simulink model "dds_cwg"  (R2016b)
(part 10 of 67)

      mask prompts: io_names "Names [msb...lsb]"; io_widths "Bitwidths [msb...lsb]"; io_bps "Binary pts [msb...lsb]"; io_types "Data types [msb...lsb], ufix=0, fix=1, bool=2"; show_format "Print format string?"; snap_storage "Storage medium"; snap_dram_dimm "DRAM dimm"; snap_dram_clock "DRAM clock rate"; snap_nsamples "Number of Samples (2^?)"; snap_data_width "Data width"; snap_offset "Start delay support"; snap_circap "Circular capture support"; snap_value "Extra value capture support"; snap_ext_arm "External arm support"; snap_ext_circ "External circular capture support"; snap_provide_outputs "Provide outputs"; snap_use_dsp48 "Use DSP48s to implement counters"; snap_delay "Pre-snapshot delay"; extra_names "Names [msb...lsb]"; extra_widths "Widths [msb...lsb]"; extra_bps "Binary pts [msb...lsb]"; extra_types "Data types [msb...lsb], ufix=0, fix=1, bool=2"
      mask help:
      | A wrapped snapshot block. Allows specification of inputs to a snapblock word so the toolflow can automatically set up the scope.
      | See documentation for snapshot for explanation of parameters.
      mask init:
      | bitsnap_init(gcb);
      settings: AttributesFormatString=|
      | snap(3):f10.9,b,b = 12 bits\n16 wide, 8192 deep
      | debugID: 72770927
      mask TypeOptions snap_storage: bram | dram
      mask Callback snap_storage: bitsnap_callback();
      mask TypeOptions snap_dram_dimm: 1 | 2 | 3 | 4
      mask TypeOptions snap_dram_clock: 200 | 250 | 266 | 300 | 333
      mask TypeOptions snap_data_width: 8 | 16 | 32 | 64 | 128
      mask Callback snap_value: bitsnap_callback();
      mask Callback snap_ext_arm: bitsnap_callback();
      mask Callback snap_ext_circ: bitsnap_callback();
      mask Callback snap_provide_outputs: bitsnap_callback();
  ss_fir_out : Subsystem  Tag=casper:bitsnap  Commented=on  AncestorBlock=casper_library_scopes/bitfield_snapshot  mask(bitsnap){io_names=[fir sync dv], io_widths=[18 1 1], io_bps=[17 0 0], io_types=[1 2 2], show_format=on, snap_storage=bram, snap_dram_dimm=2, snap_dram_clock=250, snap_nsamples=13, snap_data_width=32, snap_offset=off, snap_circap=off, snap_value=off, snap_ext_arm=off, snap_ext_circ=off, snap_provide_outputs=on, snap_use_dsp48=on, snap_delay=2, extra_names=timestamp, extra_widths=32, extra_bps=0, extra_types=0}
      mask prompts: io_names "Names [msb...lsb]"; io_widths "Bitwidths [msb...lsb]"; io_bps "Binary pts [msb...lsb]"; io_types "Data types [msb...lsb], ufix=0, fix=1, bool=2"; show_format "Print format string?"; snap_storage "Storage medium"; snap_dram_dimm "DRAM dimm"; snap_dram_clock "DRAM clock rate"; snap_nsamples "Number of Samples (2^?)"; snap_data_width "Data width"; snap_offset "Start delay support"; snap_circap "Circular capture support"; snap_value "Extra value capture support"; snap_ext_arm "External arm support"; snap_ext_circ "External circular capture support"; snap_provide_outputs "Provide outputs"; snap_use_dsp48 "Use DSP48s to implement counters"; snap_delay "Pre-snapshot delay"; extra_names "Names [msb...lsb]"; extra_widths "Widths [msb...lsb]"; extra_bps "Binary pts [msb...lsb]"; extra_types "Data types [msb...lsb], ufix=0, fix=1, bool=2"
      mask help:
      | A wrapped snapshot block. Allows specification of inputs to a snapblock word so the toolflow can automatically set up the scope.
      | See documentation for snapshot for explanation of parameters.
      mask init:
      | bitsnap_init(gcb);
      settings: AttributesFormatString=|
      | snap(3):f18.17,b,b = 20 bits\n32 wide, 8192 deep
      | debugID: 20209532
      mask TypeOptions snap_storage: bram | dram
      mask Callback snap_storage: bitsnap_callback();
      mask TypeOptions snap_dram_dimm: 1 | 2 | 3 | 4
      mask TypeOptions snap_dram_clock: 200 | 250 | 266 | 300 | 333
      mask TypeOptions snap_data_width: 8 | 16 | 32 | 64 | 128
      mask Callback snap_value: bitsnap_callback();
      mask Callback snap_ext_arm: bitsnap_callback();
      mask Callback snap_ext_circ: bitsnap_callback();
      mask Callback snap_provide_outputs: bitsnap_callback();
  ss_fir_out1 : Subsystem  Tag=casper:bitsnap  AncestorBlock=casper_library_scopes/bitfield_snapshot  mask(bitsnap){io_names=[fir sync dv], io_widths=[18 1 1], io_bps=[17 0 0], io_types=[1 2 2], show_format=on, snap_storage=bram, snap_dram_dimm=2, snap_dram_clock=250, snap_nsamples=13, snap_data_width=32, snap_offset=off, snap_circap=off, snap_value=off, snap_ext_arm=off, snap_ext_circ=off, snap_provide_outputs=on, snap_use_dsp48=on, snap_delay=2, extra_names=timestamp, extra_widths=32, extra_bps=0, extra_types=0}
      mask prompts: io_names "Names [msb...lsb]"; io_widths "Bitwidths [msb...lsb]"; io_bps "Binary pts [msb...lsb]"; io_types "Data types [msb...lsb], ufix=0, fix=1, bool=2"; show_format "Print format string?"; snap_storage "Storage medium"; snap_dram_dimm "DRAM dimm"; snap_dram_clock "DRAM clock rate"; snap_nsamples "Number of Samples (2^?)"; snap_data_width "Data width"; snap_offset "Start delay support"; snap_circap "Circular capture support"; snap_value "Extra value capture support"; snap_ext_arm "External arm support"; snap_ext_circ "External circular capture support"; snap_provide_outputs "Provide outputs"; snap_use_dsp48 "Use DSP48s to implement counters"; snap_delay "Pre-snapshot delay"; extra_names "Names [msb...lsb]"; extra_widths "Widths [msb...lsb]"; extra_bps "Binary pts [msb...lsb]"; extra_types "Data types [msb...lsb], ufix=0, fix=1, bool=2"
      mask help:
      | A wrapped snapshot block. Allows specification of inputs to a snapblock word so the toolflow can automatically set up the scope.
      | See documentation for snapshot for explanation of parameters.
      mask init:
      | bitsnap_init(gcb);
      settings: AttributesFormatString=|
      | snap(3):f18.17,b,b = 20 bits\n32 wide, 8192 deep
      | debugID: 89618929
      mask TypeOptions snap_storage: bram | dram
      mask Callback snap_storage: bitsnap_callback();
      mask TypeOptions snap_dram_dimm: 1 | 2 | 3 | 4
      mask TypeOptions snap_dram_clock: 200 | 250 | 266 | 300 | 333
      mask TypeOptions snap_data_width: 8 | 16 | 32 | 64 | 128
      mask Callback snap_value: bitsnap_callback();
      mask Callback snap_ext_arm: bitsnap_callback();
      mask Callback snap_ext_circ: bitsnap_callback();
      mask Callback snap_provide_outputs: bitsnap_callback();
  ss_nb : Subsystem  Tag=casper:bitsnap  AncestorBlock=casper_library_scopes/bitfield_snapshot  mask(bitsnap){io_names=[r0 i0 r1 i1 sync dv sync_cnt], io_widths=[18 18 18 18 1 1 11], io_bps=[17 17 17 17 0 0 0], io_types=[1 1 1 1 2 2 0], show_format=on, snap_storage=bram, snap_dram_dimm=2, snap_dram_clock=250, snap_nsamples=9, snap_data_width=128, snap_offset=off, snap_circap=off, snap_value=off, snap_ext_arm=off, snap_ext_circ=off, snap_provide_outputs=on, snap_use_dsp48=on, snap_delay=2, extra_names=timestamp, extra_widths=32, extra_bps=0, extra_types=0}
      mask prompts: io_names "Names [msb...lsb]"; io_widths "Bitwidths [msb...lsb]"; io_bps "Binary pts [msb...lsb]"; io_types "Data types [msb...lsb], ufix=0, fix=1, bool=2"; show_format "Print format string?"; snap_storage "Storage medium"; snap_dram_dimm "DRAM dimm"; snap_dram_clock "DRAM clock rate"; snap_nsamples "Number of Samples (2^?)"; snap_data_width "Data width"; snap_offset "Start delay support"; snap_circap "Circular capture support"; snap_value "Extra value capture support"; snap_ext_arm "External arm support"; snap_ext_circ "External circular capture support"; snap_provide_outputs "Provide outputs"; snap_use_dsp48 "Use DSP48s to implement counters"; snap_delay "Pre-snapshot delay"; extra_names "Names [msb...lsb]"; extra_widths "Widths [msb...lsb]"; extra_bps "Binary pts [msb...lsb]"; extra_types "Data types [msb...lsb], ufix=0, fix=1, bool=2"
      mask help:
      | A wrapped snapshot block. Allows specification of inputs to a snapblock word so the toolflow can automatically set up the scope.
      | See documentation for snapshot for explanation of parameters.
      mask init:
      | bitsnap_init(gcb);
      settings: AttributesFormatString=|
      | snap(7):f18.17,f18.17,f18.17,f18.17,b,b,uf11.0 = 85 bits\n128 wide, 512 deep
      | debugID: 83317040
      mask TypeOptions snap_storage: bram | dram
      mask Callback snap_storage: bitsnap_callback();
      mask TypeOptions snap_dram_dimm: 1 | 2 | 3 | 4
      mask TypeOptions snap_dram_clock: 200 | 250 | 266 | 300 | 333
      mask TypeOptions snap_data_width: 8 | 16 | 32 | 64 | 128
      mask Callback snap_value: bitsnap_callback();
      mask Callback snap_ext_arm: bitsnap_callback();
      mask Callback snap_ext_circ: bitsnap_callback();
      mask Callback snap_provide_outputs: bitsnap_callback();
  ss_nb1 : Subsystem  Tag=casper:bitsnap  AncestorBlock=casper_library_scopes/bitfield_snapshot  mask(bitsnap){io_names=[r2 i2 r3 i3 sync dv sync_cnt], io_widths=[18 18 18 18 1 1 11], io_bps=[17 17 17 17 0 0 0], io_types=[1 1 1 1 2 2 0], show_format=on, snap_storage=bram, snap_dram_dimm=2, snap_dram_clock=250, snap_nsamples=9, snap_data_width=128, snap_offset=off, snap_circap=off, snap_value=off, snap_ext_arm=off, snap_ext_circ=off, snap_provide_outputs=on, snap_use_dsp48=on, snap_delay=2, extra_names=timestamp, extra_widths=32, extra_bps=0, extra_types=0}
      mask prompts: io_names "Names [msb...lsb]"; io_widths "Bitwidths [msb...lsb]"; io_bps "Binary pts [msb...lsb]"; io_types "Data types [msb...lsb], ufix=0, fix=1, bool=2"; show_format "Print format string?"; snap_storage "Storage medium"; snap_dram_dimm "DRAM dimm"; snap_dram_clock "DRAM clock rate"; snap_nsamples "Number of Samples (2^?)"; snap_data_width "Data width"; snap_offset "Start delay support"; snap_circap "Circular capture support"; snap_value "Extra value capture support"; snap_ext_arm "External arm support"; snap_ext_circ "External circular capture support"; snap_provide_outputs "Provide outputs"; snap_use_dsp48 "Use DSP48s to implement counters"; snap_delay "Pre-snapshot delay"; extra_names "Names [msb...lsb]"; extra_widths "Widths [msb...lsb]"; extra_bps "Binary pts [msb...lsb]"; extra_types "Data types [msb...lsb], ufix=0, fix=1, bool=2"
      mask help:
      | A wrapped snapshot block. Allows specification of inputs to a snapblock word so the toolflow can automatically set up the scope.
      | See documentation for snapshot for explanation of parameters.
      mask init:
      | bitsnap_init(gcb);
      settings: AttributesFormatString=|
      | snap(7):f18.17,f18.17,f18.17,f18.17,b,b,uf11.0 = 85 bits\n128 wide, 512 deep
      | debugID: 32685757
      mask TypeOptions snap_storage: bram | dram
      mask Callback snap_storage: bitsnap_callback();
      mask TypeOptions snap_dram_dimm: 1 | 2 | 3 | 4
      mask TypeOptions snap_dram_clock: 200 | 250 | 266 | 300 | 333
      mask TypeOptions snap_data_width: 8 | 16 | 32 | 64 | 128
      mask Callback snap_value: bitsnap_callback();
      mask Callback snap_ext_arm: bitsnap_callback();
      mask Callback snap_ext_circ: bitsnap_callback();
      mask Callback snap_provide_outputs: bitsnap_callback();
  tlast_sel : Subsystem  Tag=xps:sw_reg  AncestorBlock=xps_library/Memory/software_register  mask(swreg){io_dir=From Processor, io_delay=0, init_val=0, sample_period=1, names=[sel], bitwidths=[1], bin_pts=0, arith_types=2, sim_port=on, show_format=on}
      mask prompts: io_dir "I/O direction"; io_delay "I/O delay"; init_val "Initial Value"; sample_period "Sample period"; names "Bitfield names [msb...lsb]"; bitwidths "Bitfield widths"; bin_pts "Bitfield binary pts"; arith_types "Bitfield types, ufix=0, fix=1, bool=2"; sim_port "Provide sim input/output?"; show_format "Print format string?"
      mask help: A 32-bit software-accessible register. Can be divided into bitfields of varying widths and types using the fields in the block mask.
      mask init:
      | swreg_init(gcb)
      settings: AttributesFormatString=1input:b = 1 bits
      mask TypeOptions io_dir: To Processor | From Processor
      mask Callback io_dir:
      | mask_enables = get_param(gcb, 'MaskEnables');
      | mask_names = get_param(gcb, 'MaskNames');
      | if strcmp(get_param(gcb, 'io_dir'), 'To Processor'),
      |     mask_enables{ismember(mask_names, 'sample_period')} = 'off';
      | else
      |     mask_enables{ismember(mask_names, 'sample_period')} = 'on';
      | end
      | set_param(gcb, 'MaskEnables', mask_enables);
      mask DialogControl ParameterTabVar0 Prompt: Setup
  tready_sel : Subsystem  Tag=xps:sw_reg  AncestorBlock=xps_library/Memory/software_register  mask(swreg){io_dir=From Processor, io_delay=0, init_val=0, sample_period=1, names=[sel], bitwidths=[1], bin_pts=0, arith_types=2, sim_port=on, show_format=on}
      mask prompts: io_dir "I/O direction"; io_delay "I/O delay"; init_val "Initial Value"; sample_period "Sample period"; names "Bitfield names [msb...lsb]"; bitwidths "Bitfield widths"; bin_pts "Bitfield binary pts"; arith_types "Bitfield types, ufix=0, fix=1, bool=2"; sim_port "Provide sim input/output?"; show_format "Print format string?"
      mask help: A 32-bit software-accessible register. Can be divided into bitfields of varying widths and types using the fields in the block mask.
      mask init:
      | swreg_init(gcb)
      settings: AttributesFormatString=1input:b = 1 bits
      mask TypeOptions io_dir: To Processor | From Processor
      mask Callback io_dir:
      | mask_enables = get_param(gcb, 'MaskEnables');
      | mask_names = get_param(gcb, 'MaskNames');
      | if strcmp(get_param(gcb, 'io_dir'), 'To Processor'),
      |     mask_enables{ismember(mask_names, 'sample_period')} = 'off';
      | else
      |     mask_enables{ismember(mask_names, 'sample_period')} = 'on';
      | end
      | set_param(gcb, 'MaskEnables', mask_enables);
      mask DialogControl ParameterTabVar0 Prompt: Setup
  tvalid_sel : Subsystem  Tag=xps:sw_reg  AncestorBlock=xps_library/Memory/software_register  mask(swreg){io_dir=From Processor, io_delay=0, init_val=0, sample_period=1, names=[sel], bitwidths=[1], bin_pts=0, arith_types=2, sim_port=on, show_format=on}
      mask prompts: io_dir "I/O direction"; io_delay "I/O delay"; init_val "Initial Value"; sample_period "Sample period"; names "Bitfield names [msb...lsb]"; bitwidths "Bitfield widths"; bin_pts "Bitfield binary pts"; arith_types "Bitfield types, ufix=0, fix=1, bool=2"; sim_port "Provide sim input/output?"; show_format "Print format string?"
      mask help: A 32-bit software-accessible register. Can be divided into bitfields of varying widths and types using the fields in the block mask.
      mask init:
      | swreg_init(gcb)
      settings: AttributesFormatString=1input:b = 1 bits
      mask TypeOptions io_dir: To Processor | From Processor
      mask Callback io_dir:
      | mask_enables = get_param(gcb, 'MaskEnables');
      | mask_names = get_param(gcb, 'MaskNames');
      | if strcmp(get_param(gcb, 'io_dir'), 'To Processor'),
      |     mask_enables{ismember(mask_names, 'sample_period')} = 'off';
      | else
      |     mask_enables{ismember(mask_names, 'sample_period')} = 'on';
      | end
      | set_param(gcb, 'MaskEnables', mask_enables);
      mask DialogControl ParameterTabVar0 Prompt: Setup
  sync_out : Outport
  pol0_out : Outport  Port=2
  pol1_out : Outport  Port=3
  dv_out : Outport  Port=4
  tag scope: capture_now=global, conf_tvalid=global, current_channel=global, data_pol0=global, data_tlast=global, data_trdy=global, fft_ch0=global, fft_ch1=global, fft_ch2=global, fft_dv0=global, fft_dv1=global, fft_dv2=global, fft_dvalid=global, fft_sync=global, fft_sync_count=global, fft_tl0=global, fft_tl1=global, fft_tl2=global, fft_tready_p0=global, fft_tready_p1=global, fft_tready_p2=global, fir_data_tlast=global, fir_dvalid_pol0=global, fir_pol0=global, fir_sync=global
  wires:
  From51/1 -> Delay13/1
  From49/1 -> Delay11/1
  Fast Fourier Transform 9.0 1/1 -> Terminator19/1
  Reinterpret1/1 -> Concat/2
  [fft_re_pol0] -> Gateway Out26/1
  Gateway Out54/1 -> To Workspace54/1
  From27/1 -> Gateway Out55/1
  Gateway Out52/1 -> To Workspace51/1
  From28/1 -> Gateway Out56/1
  pfb_fir_generic/2(pol0_out0) -> pipeline18/1(d)
  pfb_fir_generic/3(dvalid) -> pipeline19/1(d)
  pfb_fir_generic1/2(pol0_out0) -> pipeline20/1(d)
  pfb_fir_generic/1(sync_out) -> pipeline17/1(d)
  pfb_fir_generic1/1(sync_out) -> Terminator5/1
  Gateway Out56/1 -> To Workspace57/1
  Gateway Out55/1 -> To Workspace56/1
  Gateway Out26/1 -> To Workspace34/1
  Gateway Out37/1 -> To Workspace37/1
  Gateway Out38/1 -> To Workspace38/1
  pfb_fir_generic1/3(dvalid) -> pipeline21/1(d)
  [fft_fs0] -> Gateway Out54/1
  [fft_im_pol0] -> Gateway Out37/1
  Reinterpret/1 -> Concat/1
  [fft_tl0] -> Gateway Out38/1
  Reinterpret2/1 -> Concat3/1
  Reinterpret3/1 -> Concat3/2
  Concat3/1 -> Goto4/1
  Gateway Out18/1 -> To Workspace19/1
  Register11/1 -> bus_expand7/1(bus_in), Delay26/1
  Register10/1 -> Delay25/1
  Register9/1 -> Delay23/1
  Register1/1 -> bus_expand6/1(bus_in), Delay22/1
  Concat/1 -> [data_pol0]
  [capture_now] -> Register1/3
  [capture_now] -> Register9/3
  [capture_now] -> Register10/3
  [capture_now] -> Register11/3
  pipeline9/1(q) -> [fft_tl0]
  pol1/1 -> pfb_fir_generic1/2(pol0_in0)
  pipeline18/1(q) -> [fir_pol0], Gateway Out4/1
  pipeline20/1(q) -> [fir_pol1]
  Gateway Out3/1 -> To Workspace3/1
  pipeline17/1(q) -> [fir_sync], Gateway Out6/1
  Gateway Out7/1 -> To Workspace7/1
  Gateway Out16/1 -> To Workspace16/1
  [fft_sync] -> Gateway Out16/1
  pipeline8/1(q) -> [fft_dv0]
  [fft_dvalid] -> Gateway Out3/1
  [fft_tready_p0] -> Gateway Out52/1
  Gateway Out21/1 -> To Workspace21/1
  bus_expand1/1(msb_out8) -> Gateway Out21/1
  Gateway Out23/1 -> To Workspace23/1
  bus_expand1/2(out7) -> Gateway Out23/1
  Gateway Out24/1 -> To Workspace24/1
  bus_expand1/3(out6) -> Gateway Out24/1
  Gateway Out25/1 -> To Workspace27/1
  bus_expand1/4(out5) -> Gateway Out25/1
  Gateway Out28/1 -> To Workspace25/1
  bus_expand1/5(out4) -> Gateway Out28/1
  Gateway Out29/1 -> To Workspace28/1
  bus_expand1/6(out3) -> Gateway Out29/1
  Gateway Out30/1 -> To Workspace26/1
  bus_expand1/7(out2) -> Gateway Out30/1
  Gateway Out31/1 -> To Workspace29/1
  bus_expand1/8(lsb_out1) -> Gateway Out31/1
  Delay19/1 -> Register9/1
  Delay20/1 -> Register10/1
  Gateway Out6/1 -> To Workspace6/1
  Gateway Out1/1 -> To Workspace1/1
  Gateway Out4/1 -> To Workspace4/1
  Gateway Out15/1 -> To Workspace15/1
  Gateway Out33/1 -> To Workspace31/1
  Gateway Out34/1 -> To Workspace32/1
  pipeline28/1(q) -> [fft0_data_in_ch_halt]
  pipeline27/1(q) -> [fft0_event_tlast_miss]
  pipeline25/1(q) -> [fft0_event_tlast_unexp]
  [fft0_event_tlast_miss] -> Gateway Out15/1
  [fft0_event_tlast_unexp] -> Gateway Out33/1
  Gateway Out9/1 -> To Workspace9/1
  Gateway Out36/1 -> To Workspace36/1
  Gateway Out39/1 -> To Workspace39/1
  Delay3/1 -> Delay9/1
  Delay4/1 -> Delay8/1
  Gateway Out40/1 -> To Workspace40/1
  edge_detect3/1(out) -> [fft_sync]
  pipeline10/1(q) -> [fft_ch0]
  Concat5/1 -> pipeline45/1(d)
  [fft_ch] -> Gateway Out78/1, Delay12/1, Relational1/1, Delay18/1, Relational2/1
  [current_channel] -> Gateway Out34/1
  [current_channel] -> Relational/1, Delay5/1
  lsb_1/1 -> Logical6/2, Logical4/2
  lsb_0/1 -> Logical6/1, Logical4/1
  Logical4/1 -> edge_detect2/1
  [fft_dvalid] -> Delay1/1
  edge_detect2/1 -> Gateway Out40/1, [capture_now]
  [capture_now] -> Delay10/1
  Delay10/1 -> Gateway Out61/1, Delay32/1
  Register4/1 -> Concat1/4
  Register3/1 -> Concat1/3
  Register5/1 -> Concat1/2
  Register2/1 -> Concat1/1
  From1/1 -> Register2/3
  From33/1 -> Register5/3
  From34/1 -> Register3/3
  From36/1 -> Register4/3
  pipeline3/1(q) -> Register5/1
  pipeline4/1(q) -> Register3/1
  From14/1 -> Register2/2, Register5/2, Register3/2, Register4/2
  Delay13/1 -> Reinterpret3/1
  Delay11/1 -> Reinterpret2/1
  Register6/1 -> Delay16/1, Delay19/1, Delay20/1, bus_expand4/1(bus_in), Register11/1
  Delay1/1 -> Gateway Out76/1, Logical4/3
  pipeline2/1(q) -> Register2/1
  Constant/1 -> Relational/2
  Relational/1 -> Gateway Out41/1, Logical4/4
  Gateway Out41/1 -> To Workspace41/1
  pipeline44/1(q) -> [fft_fs0]
  Register12/1 -> Register4/1, pipeline4/1(d), pipeline3/1(d), pipeline2/1(d)
  From43/1 -> Register12/1
  From15/1 -> Delay7/1
  Delay7/1 -> Register12/2
  Concat1/1 -> pipeline47/1(d)
  pipeline45/1(q) -> bus_expand1/1(bus_in), pol1_out/1, bus_expand2/1(bus_in), pol0_out/1
  pipeline46/1(q) -> dv_out/1, Gateway Out18/1, pipeline80/1(d), pipeline68/1(d), pipeline82/1(d), pipeline70/1(d), Counter1/2
  pipeline19/1(q) -> Gateway Out1/1, [fir_dvalid_pol0]
  pipeline21/1(q) -> [fir_dvalid_pol1]
  pipeline26/1(q) -> [fft_tready_p0]
  pipeline13/1(q) -> [fft0_status_ch_halt]
  pipeline14/1(q) -> [fft0_data_out_ch_halt]
  Gateway Out10/1 -> To Workspace10/1
  [fft0_data_in_ch_halt] -> Gateway Out10/1
  Gateway Out11/1 -> To Workspace11/1
  [fft0_status_ch_halt] -> Gateway Out11/1
  Gateway Out42/1 -> To Workspace42/1
  [fft0_data_out_ch_halt] -> Gateway Out42/1
  Fast Fourier Transform 9.0 2/1 -> Terminator1/1
  pipeline35/1(q) -> [fft_tready_p1]
  pipeline15/1(q) -> [fft_ch1]
  pipeline50/1(q) -> [fft_dv1]
  pipeline51/1(q) -> [fft_tl1]
  pipeline34/1(q) -> [fft_tlast_unexp1]
  pipeline36/1(q) -> [fft_tlast_miss1]
  [fft_tl] -> Register13/3, Register13/1
  [fir_sync] -> Register14/3, Register14/1
  [sys_rst] -> Register15/2, Register13/2, Register14/2
  Constant10/1 -> Relational1/2
  Logical1/1 -> Register15/3, Register15/1
  Register15/1 -> Inverter1/1, Gateway Out20/1, edge_detect3/1(in)
  Delay6/1 -> [current_channel]
  Delay8/1 -> Reinterpret1/1
  Delay9/1 -> Reinterpret/1
  Logical2/1 -> Delay2/1
  Gateway Out20/1 -> To Workspace20/1
  Register13/1 -> Logical1/2
  Register14/1 -> Logical1/1
  Delay18/1 -> Relational2/2
  Relational2/1 -> Gateway Out80/1, Logical2/2
  [fft_dv] -> Delay15/1
  [capture_now] -> Gateway Out74/1, Counter/2
  Constant11/1 -> Relational3/2
  Counter/1 -> pipeline33/1(d), Gateway Out17/1, Relational3/1
  Gateway Out17/1 -> To Workspace17/1
  Gateway Out19/1 -> To Workspace18/1
  [sys_rst] -> Register8/2
  Register7/1 -> edge_detect4/1(in), Gateway Out32/1
  Gateway Out22/1 -> To Workspace22/1
  Gateway Out27/1 -> To Workspace30/1
  Gateway Out32/1 -> To Workspace33/1
  Relational3/1 -> Gateway Out19/1, Logical5/2
  Register8/1 -> pipeline114/1(d), pipeline111/1(d), Delay14/1
  Logical5/1 -> Register7/1, Gateway Out27/1, Register7/3
  [sys_rst] -> Register7/2
  [sys_rst] -> Counter1/1
  Counter1/1 -> pipeline81/1(d), pipeline69/1(d)
  [sys_rst] -> Counter2/1
  Logical3/1 -> edge_detect5/1(in)
  Gateway Out43/1 -> To Workspace43/1
  Counter2/1 -> [fft_sync_count], Gateway Out43/1
  Inverter1/1 -> Logical3/2
  Relational1/1 -> Logical3/1, Logical1/3
  edge_detect5/1(out) -> Counter2/2
  sync/1 -> Gateway Out9/1, pfb_fir_generic/1(sync), pfb_fir_generic1/1(sync), pipeline29/1(d), pipeline54/1(d)
  From54/1 -> pipeline55/1(d)
  From53/1 -> pipeline58/1(d)
  From55/1 -> pipeline64/1(d), pipeline59/1(d)
  From56/1 -> pipeline60/1(d)
  From57/1 -> pipeline63/1(d)
  From50/1 -> pipeline56/1(d)
  From52/1 -> pipeline57/1(d)
  From58/1 -> pipeline61/1(d)
  From59/1 -> pipeline62/1(d)
  pipeline55/1(q) -> ss_fft0/1(in_fft_ch)
  pipeline56/1(q) -> ss_fft0/2(in_fft_re)
  pipeline57/1(q) -> ss_fft0/3(in_fft_im)
  pipeline58/1(q) -> ss_fft0/4(in_fft_sync_cnt)
  pipeline59/1(q) -> ss_fft0/5(in_fft_dv)
  pipeline60/1(q) -> ss_fft0/7(in_fft_tl)
  pipeline61/1(q) -> ss_fft0/8(in_fft_sync)
  pipeline62/1(q) -> ss_fft0/9(in_fft_dvalid)
  pipeline63/1(q) -> ss_fft0/14(in_fir_sync)
  pipeline64/1(q) -> ss_fft0/15(we)
  pipeline65/1(q) -> ss_fft0/16(trig)
  From45/1 -> edge_detect1/1(in)
  pipeline66/1(q) -> ss_fft0/6(in_fft_fs)
  From65/1 -> pipeline66/1(d)
  edge_detect1/1(out) -> pipeline65/1(d)
  Delay14/1 -> Logical5/1, Gateway Out22/1
  edge_detect4/1(out) -> pipeline113/1(d), pipeline1/1(d)
  pipeline67/1(q) -> ss_nb/5(in_sync)
  pipeline68/1(q) -> ss_nb/6(in_dv)
  pipeline69/1(q) -> ss_nb/7(in_sync_cnt)
  pipeline70/1(q) -> ss_nb/8(we)
  pipeline71/1(q) -> ss_nb/9(trig)
  pipeline53/1(q) -> ss_fir_in/4(we)
  pipeline54/1(q) -> ss_fir_in/5(trig)
  From66/1 -> pipeline76/1(d), pipeline73/1(d)
  From67/1 -> pipeline72/1(d)
  From68/1 -> pipeline75/1(d), pipeline74/1(d)
  pipeline75/1(q) -> ss_fir_out/4(we)
  pipeline76/1(q) -> ss_fir_out/5(trig)
  [fir_sync] -> pipeline43/1(d)
  [fir_pol0] -> pipeline12/1(d)
  [fir_dvalid_pol0] -> pipeline77/1(d), pipeline52/1(d)
  pipeline77/1(q) -> ss_fir_out1/4(we)
  pipeline78/1(q) -> ss_fir_out1/5(trig)
  [fir_sync] -> Logical/1, Counter3/1
  [fir_dvalid_pol0] -> Counter3/2
  Logical/1 -> pipeline78/1(d)
  Relational4/1 -> [fir_data_tlast], Logical/2
  Counter3/1 -> Relational4/1
  Constant9/1 -> Relational4/2
  pipeline29/1(q) -> ss_fir_in/2(in_sync)
  pipeline48/1(q) -> ss_fir_in/3(in_dv)
  pipeline72/1(q) -> ss_fir_out/1(in_fir)
  pipeline73/1(q) -> ss_fir_out/2(in_sync)
  pipeline74/1(q) -> ss_fir_out/3(in_dv)
  pipeline11/1(q) -> ss_fir_in/1(in_fir)
  pipeline12/1(q) -> ss_fir_out1/1(in_fir)
  pipeline43/1(q) -> ss_fir_out1/2(in_sync)
  pipeline52/1(q) -> ss_fir_out1/3(in_dv)
  bus_expand2/1(msb_out8) -> pipeline87/1(d)
  bus_expand2/2(out7) -> pipeline86/1(d)
  bus_expand2/3(out6) -> pipeline85/1(d)
  bus_expand2/4(out5) -> pipeline84/1(d)
  pipeline84/1(q) -> ss_nb/4(in_i1)
  pipeline85/1(q) -> ss_nb/3(in_r1)
  pipeline86/1(q) -> ss_nb/2(in_i0)
  pipeline87/1(q) -> ss_nb/1(in_r0)
  pipeline79/1(q) -> ss_nb1/5(in_sync)
  pipeline80/1(q) -> ss_nb1/6(in_dv)
  pipeline81/1(q) -> ss_nb1/7(in_sync_cnt)
  pipeline82/1(q) -> ss_nb1/8(we)
  pipeline83/1(q) -> ss_nb1/9(trig)
  bus_expand2/5(out4) -> pipeline91/1(d)
  bus_expand2/6(out3) -> pipeline90/1(d)
  bus_expand2/7(out2) -> pipeline89/1(d)
  bus_expand2/8(lsb_out1) -> pipeline88/1(d)
  pipeline38/1(q) -> [fft_fs1]
  From85/1 -> pipeline92/1(d)
  From86/1 -> pipeline95/1(d), pipeline101/1(d)
  From81/1 -> pipeline100/1(d)
  From75/1 -> pipeline93/1(d)
  From78/1 -> pipeline94/1(d)
  pipeline92/1(q) -> ss_fft1/1(in_fft_ch)
  pipeline93/1(q) -> ss_fft1/2(in_fft_re)
  pipeline94/1(q) -> ss_fft1/3(in_fft_im)
  pipeline101/1(q) -> ss_fft1/13(we)
  pipeline102/1(q) -> ss_fft1/14(trig)
  From74/1 -> edge_detect6/1(in)
  edge_detect6/1(out) -> pipeline102/1(d)
  pipeline95/1(q) -> ss_fft1/4(in_fft_dv)
  From88/1 -> pipeline96/1(d)
  From87/1 -> pipeline103/1(d)
  From82/1 -> pipeline97/1(d)
  Constant2/1 -> pipeline98/1(d)
  pipeline98/1(q) -> ss_fft1/8(in_fft_of)
  pipeline97/1(q) -> ss_fft1/7(in_fft_sync)
  pipeline103/1(q) -> ss_fft1/6(in_fft_tl)
  pipeline96/1(q) -> ss_fft1/5(in_fft_fs)
  pipeline100/1(q) -> ss_fft1/12(in_fir_sync)
  From76/1 -> pipeline99/1(d)
  pipeline99/1(q) -> ss_fft1/9(in_fft_tready)
  pipeline104/1(q) -> ss_fft0/11(in_fft_tready)
  pipeline105/1(q) -> ss_fft0/10(in_fft_of)
  From77/1 -> pipeline104/1(d)
  Constant1/1 -> pipeline105/1(d)
  Fast Fourier Transform 9.0 3/1 -> Terminator6/1
  Fast Fourier Transform 9.0 3/2 -> pipeline117/1(d)
  dvalid/1 -> Fast Fourier Transform 9.0 2/5, Gateway Out36/1, pfb_fir_generic1/3(en), pfb_fir_generic/3(en), pipeline48/1(d), pipeline53/1(d)
  pipeline117/1(q) -> [fft_tready_p2]
  pipeline110/1(q) -> [fft_ch2]
  pipeline124/1(q) -> [fft_dv2]
  pipeline125/1(q) -> [fft_tl2]
  pipeline116/1(q) -> [fft_tlast_unexp2]
  pipeline120/1(q) -> [fft_fs2]
  From98/1 -> pipeline126/1(d)
  From94/1 -> pipeline107/1(d), pipeline129/1(d)
  From92/1 -> pipeline106/1(d)
  pipeline126/1(q) -> ss_fft2/1(in_fft_ch)
  pipeline127/1(q) -> ss_fft2/2(in_fft_re)
  pipeline128/1(q) -> ss_fft2/3(in_fft_im)
  pipeline107/1(q) -> ss_fft2/13(we)
  pipeline108/1(q) -> ss_fft2/14(trig)
  From83/1 -> edge_detect7/1(in)
  edge_detect7/1(out) -> pipeline108/1(d)
  pipeline129/1(q) -> ss_fft2/4(in_fft_dv)
  From95/1 -> pipeline130/1(d)
  From96/1 -> pipeline109/1(d)
  From93/1 -> pipeline131/1(d)
  Constant3/1 -> pipeline132/1(d)
  pipeline132/1(q) -> ss_fft2/8(in_fft_of)
  pipeline131/1(q) -> ss_fft2/7(in_fft_sync)
  pipeline109/1(q) -> ss_fft2/6(in_fft_tl)
  pipeline130/1(q) -> ss_fft2/5(in_fft_fs)
  pipeline106/1(q) -> ss_fft2/12(in_fir_sync)
  From89/1 -> pipeline133/1(d)
  pipeline133/1(q) -> ss_fft2/9(in_fft_tready)
  Gateway Out35/1 -> To Workspace35/1
  [fir_data_tlast] -> Gateway Out35/1
  Constant28/1 -> data_tready/1(sim_1)
  pipeline134/1(q) -> ss_fft2/10(in_tlast_miss)
  pipeline118/1(q) -> [fft_tlast_miss2]
  From102/1 -> pipeline134/1(d)
  pipeline135/1(q) -> ss_fft1/10(in_tlast_miss)
  From103/1 -> pipeline135/1(d)
  pipeline136/1(q) -> ss_fft1/11(in_tlast_unexp)
  From104/1 -> pipeline136/1(d)
  pipeline137/1(q) -> ss_fft2/11(in_tlast_unexp)
  From105/1 -> pipeline137/1(d)
  pipeline138/1(q) -> ss_fft0/13(in_tlast_unexp)
  pipeline139/1(q) -> ss_fft0/12(in_tlast_miss)
  From106/1 -> pipeline138/1(d)
  From107/1 -> pipeline139/1(d)
  Gateway Out44/1 -> To Workspace72/1
  [fft0_event_tlast_unexp] -> Gateway Out44/1
  Gateway Out45/1 -> To Workspace44/1
  [fft0_event_tlast_miss] -> Gateway Out45/1
  Gateway Out47/1 -> To Workspace47/1
  [fft_tlast_unexp1] -> Gateway Out47/1
  Gateway Out48/1 -> To Workspace48/1
  [fft_tlast_miss1] -> Gateway Out48/1
  Gateway Out50/1 -> To Workspace50/1
  Gateway Out51/1 -> To Workspace52/1
  Gateway Out53/1 -> To Workspace53/1
  [fft_ch1] -> Gateway Out50/1
  [fft_dv1] -> Gateway Out51/1
  [fft_tl1] -> Gateway Out53/1
  Gateway Out57/1 -> To Workspace55/1
  [fft_fs1] -> Gateway Out57/1
  Gateway Out58/1 -> To Workspace58/1
  [fft_re_pol1] -> Gateway Out58/1
  Gateway Out59/1 -> To Workspace59/1
  [fft_im_pol1] -> Gateway Out59/1
  Gateway Out60/1 -> To Workspace60/1
  [fft_tready_p1] -> Gateway Out60/1
  Gateway Out62/1 -> To Workspace62/1
  [fft_dv0] -> Gateway Out62/1
  Gateway Out63/1 -> To Workspace61/1
  Gateway Out64/1 -> To Workspace63/1
  Gateway Out66/1 -> To Workspace65/1
  Gateway Out67/1 -> To Workspace66/1
  Gateway Out68/1 -> To Workspace67/1
  Gateway Out69/1 -> To Workspace68/1
  Gateway Out70/1 -> To Workspace69/1
  Gateway Out71/1 -> To Workspace70/1
  Gateway Out72/1 -> To Workspace71/1
  [fft_fs2] -> Gateway Out69/1
  [fft_tlast_unexp2] -> Gateway Out63/1
  [fft_tlast_miss2] -> Gateway Out64/1
  [fft_tl2] -> Gateway Out68/1
  [fft_dv2] -> Gateway Out67/1
  [fft_ch2] -> Gateway Out66/1
  [fft_re_pol2] -> Gateway Out70/1
  [fft_im_pol2] -> Gateway Out71/1
  [fft_tready_p2] -> Gateway Out72/1
  Fast Fourier Transform 9.0 3/3 -> pipeline122/1(d)
  Fast Fourier Transform 9.0 3/4 -> pipeline123/1(d)
  Fast Fourier Transform 9.0 3/5 -> pipeline110/1(d)
  Fast Fourier Transform 9.0 3/6 -> pipeline124/1(d)
  Fast Fourier Transform 9.0 3/7 -> pipeline125/1(d)
  Fast Fourier Transform 9.0 3/8 -> pipeline120/1(d)
  Fast Fourier Transform 9.0 3/9 -> pipeline116/1(d)
  Fast Fourier Transform 9.0 3/10 -> pipeline118/1(d)
  Fast Fourier Transform 9.0 3/11 -> Terminator7/1
  Fast Fourier Transform 9.0 3/12 -> Terminator8/1
  Fast Fourier Transform 9.0 3/13 -> Terminator9/1
  pipeline122/1(q) -> [fft_im_pol2]
  pipeline123/1(q) -> [fft_re_pol2]
  [fft_fwd_inv] -> Fast Fourier Transform 9.0 2/1
  Constant6/1 -> Fast Fourier Transform 9.0 2/3
  pol0/1 -> Fast Fourier Transform 9.0 2/4, pipeline11/1(d), Gateway Out39/1, pfb_fir_generic/2(pol0_in0)
  Fast Fourier Transform 9.0 2/2 -> pipeline35/1(d)
  Fast Fourier Transform 9.0 2/3 -> pipeline40/1(d)
  Fast Fourier Transform 9.0 2/4 -> pipeline49/1(d)
  Fast Fourier Transform 9.0 2/6 -> pipeline50/1(d)
  Fast Fourier Transform 9.0 2/5 -> pipeline15/1(d)
  Fast Fourier Transform 9.0 2/7 -> pipeline51/1(d)
  Fast Fourier Transform 9.0 2/8 -> pipeline38/1(d)
  Fast Fourier Transform 9.0 2/9 -> pipeline34/1(d)
  Fast Fourier Transform 9.0 2/10 -> pipeline36/1(d)
  Fast Fourier Transform 9.0 2/11 -> Terminator2/1
  pipeline40/1(q) -> [fft_im_pol1]
  pipeline49/1(q) -> [fft_re_pol1]
  From84/1 -> pipeline127/1(d)
  From90/1 -> pipeline128/1(d)
  [fft_fwd_inv] -> Fast Fourier Transform 9.0 3/2
  [fir_dvalid_pol0] -> Fast Fourier Transform 9.0 3/6
  [fir_pol0] -> Fast Fourier Transform 9.0 3/5
  Constant18/1 -> Fast Fourier Transform 9.0 3/4
  [fir_sync] -> edge_detect8/1(in)
  [fft_scale] -> Fast Fourier Transform 9.0 3/1
  [fft_fwd_inv] -> Fast Fourier Transform 9.0 1/1
  Constant7/1 -> Fast Fourier Transform 9.0 1/3
  [fir_pol0] -> Fast Fourier Transform 9.0 1/4
  [fir_dvalid_pol0] -> Fast Fourier Transform 9.0 1/5
  [data_tlast] -> Fast Fourier Transform 9.0 1/6
  Fast Fourier Transform 9.0 1/2 -> pipeline26/1(d)
  Fast Fourier Transform 9.0 1/3 -> pipeline6/1(d)
  Fast Fourier Transform 9.0 1/4 -> pipeline7/1(d)
  Fast Fourier Transform 9.0 1/5 -> pipeline10/1(d)
  Fast Fourier Transform 9.0 1/6 -> pipeline8/1(d)
  Fast Fourier Transform 9.0 1/7 -> pipeline9/1(d)
  Fast Fourier Transform 9.0 1/8 -> pipeline44/1(d)
  Fast Fourier Transform 9.0 1/9 -> pipeline25/1(d)
  Fast Fourier Transform 9.0 1/10 -> pipeline27/1(d)
  Fast Fourier Transform 9.0 1/11 -> pipeline28/1(d)
  Fast Fourier Transform 9.0 1/12 -> pipeline13/1(d)
  Fast Fourier Transform 9.0 1/13 -> pipeline14/1(d)
  pipeline7/1(q) -> [fft_re_pol0]
  pipeline6/1(q) -> [fft_im_pol0]
  Fast Fourier Transform 9.0 2/12 -> Terminator3/1
  Fast Fourier Transform 9.0 2/13 -> Terminator4/1
  [conf_tvalid] -> Fast Fourier Transform 9.0 1/2
  edge_detect8/1(out) -> Mux/2
  data_tready/1(in_rdy) -> pipeline234/1(d)
  Constant13/1 -> tvalid_sel/1(sim_1)
  tvalid_sel/1(in_sel) -> pipeline5/1(d)
  Constant14/1 -> conf_tvalid/1(sim_1)
  conf_tvalid/1(in_tvalid) -> pipeline16/1(d)
  pipeline5/1(q) -> Mux/1
  pipeline16/1(q) -> Mux/3
  Mux/1 -> [conf_tvalid]
  [conf_tvalid] -> Fast Fourier Transform 9.0 3/3
  [data_trdy] -> Fast Fourier Transform 9.0 3/8
  [data_trdy] -> Fast Fourier Transform 9.0 2/7
  [data_trdy] -> Fast Fourier Transform 9.0 1/7
  pipeline234/1(q) -> Mux1/3
  Mux1/1 -> [data_trdy]
  Constant8/1 -> Mux1/2
  Constant12/1 -> tready_sel/1(sim_1)
  tready_sel/1(in_sel) -> pipeline22/1(d)
  pipeline22/1(q) -> Mux1/1
  [conf_tvalid] -> Fast Fourier Transform 9.0 2/2
  Constant15/1 -> data_tlast/1(sim_1)
  data_tlast/1(in_rdy) -> pipeline24/1(d)
  Constant4/1 -> tlast_sel/1(sim_1)
  tlast_sel/1(in_sel) -> pipeline23/1(d)
  pipeline23/1(q) -> Mux2/1
  pipeline24/1(q) -> Mux2/2
  [fir_data_tlast] -> Mux2/3
  Mux2/1 -> [data_tlast]
  [data_tlast] -> Fast Fourier Transform 9.0 3/7
  [data_tlast] -> Fast Fourier Transform 9.0 2/6
  [fft_re_pol0] -> Mux3/2
  [fft_re_pol2] -> Mux3/4
  [fft_re_pol1] -> Convert2/1
  [fft_im_pol0] -> Mux4/2
  [fft_im_pol1] -> Convert3/1
  [fft_im_pol2] -> Mux4/4
  Constant5/1 -> data_sel/1(sim_1)
  pipeline30/1(q) -> Mux3/1
  pipeline31/1(q) -> Mux4/1
  Mux3/1 -> Delay3/1
  Mux4/1 -> Delay4/1
  Convert2/1 -> Mux3/3
  Convert3/1 -> Mux4/3
  pipeline88/1(q) -> ss_nb1/4(in_i3)
  pipeline89/1(q) -> ss_nb1/3(in_r3)
  pipeline90/1(q) -> ss_nb1/2(in_i2)
  pipeline91/1(q) -> ss_nb1/1(in_r2)
  pipeline115/1(q) -> ss_cap/1(in_sync)
  pipeline32/1(q) -> ss_cap/3(in_cap_now)
  pipeline33/1(q) -> ss_cap/4(in_cap_cntr)
  pipeline37/1(q) -> ss_cap/5(in_r0)
  pipeline39/1(q) -> ss_cap/6(in_i0)
  pipeline111/1(q) -> ss_cap/8(we)
  pipeline112/1(q) -> ss_cap/9(trig)
  pipeline113/1(q) -> ss_cap/7(in_sync_out)
  From139/1 -> pipeline32/1(d)
  bus_expand5/1(msb_out2) -> Gateway Out46/1, pipeline37/1(d)
  bus_expand5/2(lsb_out1) -> Gateway Out49/1, pipeline39/1(d)
  pipeline114/1(q) -> ss_cap/2(in_dv)
  [data_pol0] -> bus_expand3/1(bus_in)
  Gateway Out2/1 -> To Workspace2/1
  Gateway Out5/1 -> To Workspace5/1
  bus_expand3/1(msb_out2) -> Gateway Out2/1
  bus_expand3/2(lsb_out1) -> Gateway Out5/1
  Gateway Out8/1 -> To Workspace8/1
  [fft_ch0] -> Gateway Out8/1
  data_sel/1(in_sel) -> pipeline140/1(d), pipeline121/1(d), pipeline119/1(d), pipeline31/1(d), pipeline30/1(d)
  pipeline119/1(q) -> Mux5/1
  [fft_ch2] -> Mux5/4
  [fft_ch1] -> Mux5/3
  [fft_ch0] -> Mux5/2
  pipeline121/1(q) -> Mux6/1
  [fft_dv2] -> Mux6/4
  [fft_dv1] -> Mux6/3
  [fft_dv0] -> Mux6/2
  Mux6/1 -> [fft_dv]
  Mux5/1 -> [fft_ch]
  pipeline140/1(q) -> Mux7/1
  [fft_tl2] -> Mux7/4
  [fft_tl1] -> Mux7/3
  [fft_tl0] -> Mux7/2
  Mux7/1 -> [fft_tl]
  Delay16/1 -> bus_expand5/1(bus_in), Register1/1
  Gateway Out12/1 -> To Workspace12/1
  [fft_sync] -> Gateway Out75/1, pipeline115/1(d), pipeline112/1(d), Register8/1, Register8/3, Counter/1
  Delay24/1 -> Register1/2, Register11/2, Register10/2, Register9/2
  Gateway Out13/1 -> To Workspace13/1
  bus_expand4/1(msb_out2) -> Gateway Out13/1
  Gateway Out14/1 -> To Workspace14/1
  bus_expand4/2(lsb_out1) -> Gateway Out14/1
  Gateway Out46/1 -> To Workspace45/1
  Gateway Out49/1 -> To Workspace46/1
  Delay22/1 -> Delay27/1
  Delay23/1 -> Delay28/1
  Delay25/1 -> Delay29/1
  Delay26/1 -> Delay30/1
  Delay27/1 -> Concat5/1
  Delay28/1 -> Concat5/2
  Delay29/1 -> Concat5/3
  Delay30/1 -> Concat5/4
  Delay31/1 -> pipeline46/1(d)
  Delay32/1 -> Delay31/1
  pipeline1/1(q) -> pipeline83/1(d), pipeline71/1(d), pipeline79/1(d), pipeline67/1(d), Gateway Out7/1, sync_out/1
  Gateway Out61/1 -> To Workspace49/1
  [data_pol0] -> Register6/1
  [fft_dvalid] -> Register6/2
  [fft_sync] -> Delay24/1
  bus_expand6/1(msb_out2) -> To Workspace64/1
  bus_expand6/2(lsb_out1) -> To Workspace73/1
  Gateway Out65/1 -> To Workspace74/1
  bus_expand7/1(msb_out2) -> Gateway Out65/1
  Gateway Out73/1 -> To Workspace75/1
  bus_expand7/2(lsb_out1) -> Gateway Out73/1
  Gateway Out74/1 -> To Workspace76/1
  Gateway Out75/1 -> To Workspace77/1
  Gateway Out76/1 -> To Workspace78/1
  Gateway Out77/1 -> To Workspace79/1
  Logical6/1 -> Gateway Out77/1
  Delay2/1 -> [fft_dvalid]
  Gateway Out78/1 -> To Workspace80/1
  Gateway Out79/1 -> To Workspace81/1
  Gateway Out80/1 -> To Workspace82/1
  Gateway Out81/1 -> To Workspace83/1
  Delay17/1 -> Gateway Out81/1, Delay6/1
  Delay12/1 -> Delay17/1
  Delay15/1 -> Delay21/1
  Delay21/1 -> Gateway Out79/1, Logical2/1
  Delay5/1 -> Delay33/1, Gateway Out12/1, lsb_1/1, lsb_0/1
  Delay33/1 -> Delay34/1
  Delay34/1 -> Delay35/1
  Delay35/1 -> pipeline41/1(d)
  Gateway Out82/1 -> To Workspace84/1
  pipeline41/1(q) -> Gateway Out82/1
